simulink model "P4"  (R2020b)
settings: Solver=VariableStepAuto  StartTime=0.0  StopTime=10.0  RelTol=1e-3
settings Model: Creator=stank  LastModifiedBy=stank

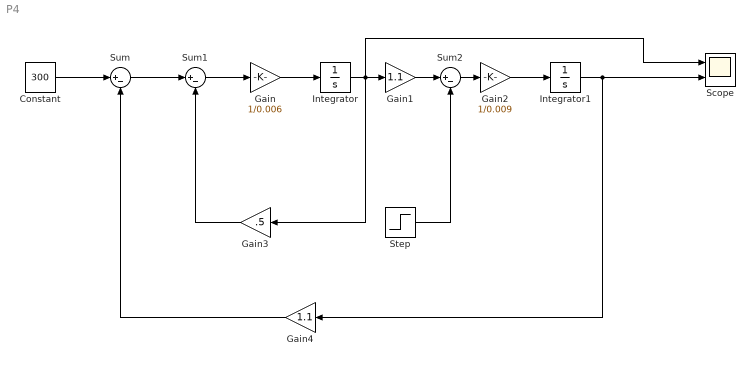
== system P4 ==
  Constant : Constant  Value=300
  Gain : Gain  Gain=1/0.006
  Gain1 : Gain  Gain=1.1
  Gain2 : Gain  Gain=1/0.009
  Gain3 : Gain  Gain=.5
  Gain4 : Gain  Gain=1.1
  Integrator : Integrator
  Integrator1 : Integrator
  Scope : Scope  NumInputPorts=2
  Step : Step  SampleTime=0
  Sum : Sum  Inputs=|+-
  Sum1 : Sum  Inputs=|+-
  Sum2 : Sum  Inputs=|+-
  wires:
  Constant/1 -> Sum/1
  Sum/1 -> Sum1/1
  Sum1/1 -> Gain/1
  Gain/1 -> Integrator/1
  Gain1/1 -> Sum2/1
  Sum2/1 -> Gain2/1
  Gain2/1 -> Integrator1/1
  Integrator1/1 -> Gain4/1, Scope/2
  Gain4/1 -> Sum/2
  Gain3/1 -> Sum1/2
  Step/1 -> Sum2/2
  Integrator/1 -> Gain3/1, Scope/1, Gain1/1
